simulink model "model"  (R2017a)
settings: Solver=ode45  StartTime=0.0  StopTime=2  RelTol=1e-3  EnableMultiTasking=on
undefined symbols (not defined in the file or in its folder): current_ctrl, motor, vest
libraries: simulink x1
settings Model: Creator=rodrigo  LastModifiedBy=rodrigo
settings DataIOCC: LimitDataPoints=on  SaveFormat=Array
settings OptimizationCC: LifeSpan=inf
settings DebuggingCC: UnderspecifiedInitializationDetection=Classic  MergeDetectMultiDrivingBlocksExec=none  StateNameClashWarn=warning  SFUnexpectedBacktrackingDiag=warning  SFNoUnconditionalDefaultTransitionDiag=warning  SFExecutionAtInitializationDiag=none
settings HardwareCC: ProdBitPerPointer=32  ProdBitPerSizeT=32  ProdBitPerPtrDiffT=32  ProdLargestAtomicFloat=None  ProdIntDivRoundTo=Undefined  ProdEndianess=Unspecified  ProdWordSize=32  ProdHWDeviceType=32-bit Generic
settings ModelReferenceCC: PropagateSignalLabelsOutOfModel=off
settings GRTTargetCC: TargetLangStandard=C89/C90 (ANSI)  GeneratePreprocessorConditionals=Disable all
settings ConfigComp: CovMetricSettings=dw  CovHtmlReporting=on  CovSaveCumulativeToWorkspaceVar=on  CovSaveSingleToWorkspaceVar=on  CovExternalEMLEnable=off

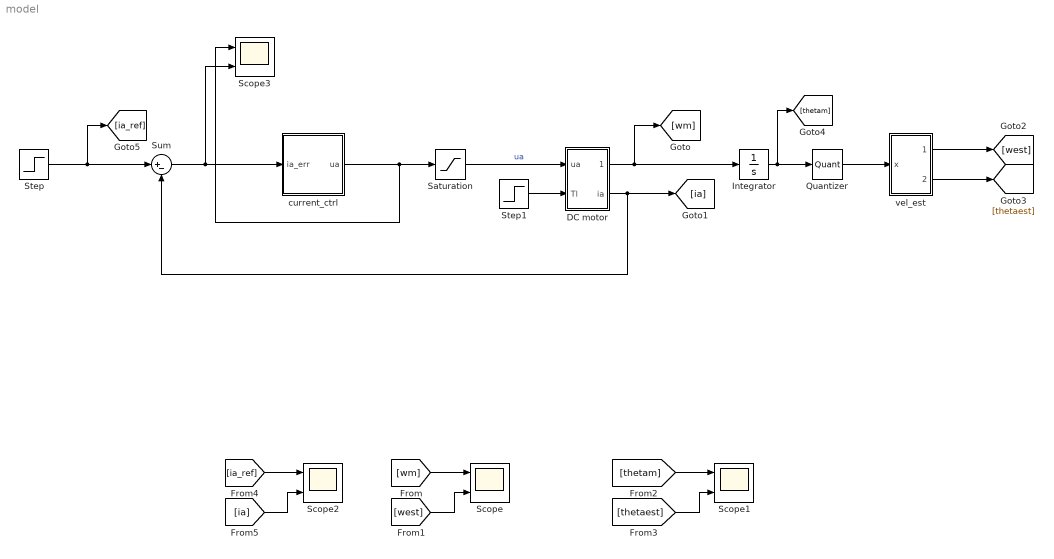
== system model ==
  DC motor : Subsystem
  Integrator : Integrator
  Quantizer : Quantizer  QuantizationInterval=encoder
  Saturation : Saturate  UpperLimit=12  LowerLimit=-12
  Scope{,1..3} (4 alike) : Scope  NumInputPorts=2
  Step : Step  Time=0.1  After=0.5  SampleTime=0
  Step1 : Step  Time=0.6  After=0.05  SampleTime=0  ZeroCross=off
  Sum : Sum  Inputs=|+-
  current_ctrl : Subsystem
  vel_est : Subsystem
  wires:
  Step/1 -> [ia_ref], Sum/1
  [wm] -> Scope/1
  [west] -> Scope/2
  DC motor/2(ia) -> [ia], Sum/2
  Step1/1 -> DC motor/2(Tl)
  Saturation/1 -> DC motor/1(ua)  "ua"
  DC motor/1(wm) -> Integrator/1, [wm]
  Integrator/1 -> [thetam], Quantizer/1
  Quantizer/1 -> vel_est/1(x)
  vel_est/1(vest) -> [west]
  [thetam] -> Scope1/1
  [thetaest] -> Scope1/2
  vel_est/2(xest) -> [thetaest]
  [ia_ref] -> Scope2/1
  [ia] -> Scope2/2
  Sum/1 -> Scope3/2, current_ctrl/1(ia_err)
  current_ctrl/1(ua) -> Scope3/1, Saturation/1

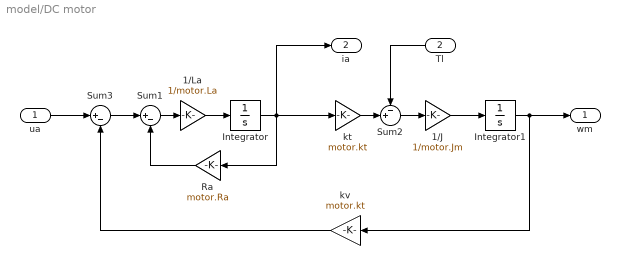
== system model/DC motor ==
  ua : Inport
  Tl : Inport  Port=2
  1/J : Gain  Gain=1/motor.Jm
  1/La : Gain  Gain=1/motor.La
  Integrator : Integrator  ZeroCross=off
  Integrator1 : Integrator
  Ra : Gain  Gain=motor.Ra
  Sum1 : Sum  Inputs=|+-
  Sum2 : Sum  Inputs=-+|
  Sum3 : Sum  Inputs=|+-
  kt : Gain  Gain=motor.kt
  kv : Gain  Gain=motor.kt
  wm : Outport
  ia : Outport  Port=2
  wires:
  1/J/1 -> Integrator1/1
  Sum2/1 -> 1/J/1
  Integrator1/1 -> wm/1, kv/1
  ua/1 -> Sum3/1
  Integrator/1 -> kt/1, Ra/1, ia/1
  Ra/1 -> Sum1/2
  1/La/1 -> Integrator/1
  Tl/1 -> Sum2/1
  kv/1 -> Sum3/2
  Sum3/1 -> Sum1/1
  kt/1 -> Sum2/2
  Sum1/1 -> 1/La/1

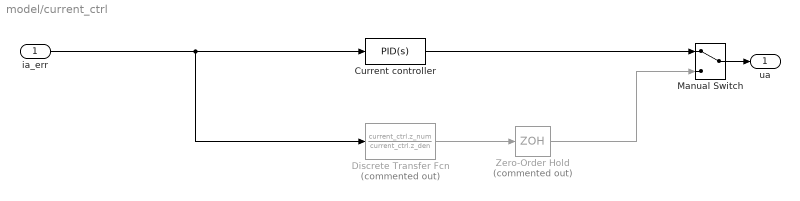
== system model/current_ctrl ==
  ia_err : Inport
  Current controller : simulink/Continuous/PID Controller  Controller=PID  TimeDomain=Continuous-time  SampleTime=-1  IntegratorMethod=Forward Euler  FilterMethod=Forward Euler  Form=Parallel  UseFilter=off  ControllerParametersSource=internal  P=current_ctrl.kp  I=current_ctrl.ki  D=0  N=100  InitialConditionSource=internal  InitialConditionForIntegrator=0  InitialConditionForFilter=0  ExternalReset=none  ZeroCross=off  LimitOutput=on  UpperSaturationLimit=12  LowerSaturationLimit=-12  LinearizeAsGain=off  AntiWindupMode=back-calculation  Kb=1  TrackingMode=off  Kt=1  PParamMin=[]  PParamMax=[]  IParamMin=[]  IParamMax=[]  DParamMin=[]  DParamMax=[]  NParamMin=[]  NParamMax=[]  KbParamMin=[]  KbParamMax=[]  KtParamMin=[]  KtParamMax=[]  POutMin=[]  POutMax=[]  IOutMin=[]  IOutMax=[]  DOutMin=[]  DOutMax=[]  NOutMin=[]  NOutMax=[]  KbOutMin=[]  KbOutMax=[]  KtOutMin=[]  KtOutMax=[]  IntegratorOutMin=[]  IntegratorOutMax=[]  FilterOutMin=[]  FilterOutMax=[]  SumOutMin=[]  SumOutMax=[]  SumI1OutMin=[]  SumI1OutMax=[]  SumI2OutMin=[]  SumI2OutMax=[]  SumI3OutMin=[]  SumI3OutMax=[]  SumDOutMin=[]  SumDOutMax=[]  SaturationOutMin=[]  SaturationOutMax=[]  IntegratorContinuousStateAttributes=''  IntegratorStateMustResolveToSignalObject=off  IntegratorRTWStateStorageClass=Auto  FilterContinuousStateAttributes=''  FilterStateMustResolveToSignalObject=off  FilterRTWStateStorageClass=Auto  DifferentiatorICPrevScaledInput=0  DifferentiatorOutMin=[]  DifferentiatorOutMax=[]  InitialConditionSetting=State (most efficient)
  Discrete Transfer Fcn : DiscreteTransferFcn  Commented=on  Numerator=current_ctrl.z_num  Denominator=current_ctrl.z_den  SampleTime=current_ctrl.Ts
  Manual Switch : ManualSwitch
  Zero-Order Hold : ZeroOrderHold  Commented=on  SampleTime=-1
  ua : Outport
  wires:
  ia_err/1 -> Discrete Transfer Fcn/1, Current controller/1
  Current controller/1 -> Manual Switch/1
  Discrete Transfer Fcn/1 -> Zero-Order Hold/1
  Zero-Order Hold/1 -> Manual Switch/2
  Manual Switch/1 -> ua/1

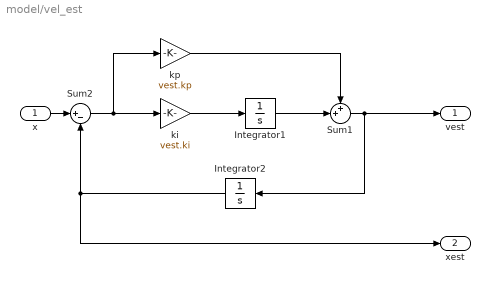
== system model/vel_est ==
  x : Inport
  Integrator1 : Integrator
  Integrator2 : Integrator
  Sum1 : Sum  Inputs=++|
  Sum2 : Sum  Inputs=|+-
  ki : Gain  Gain=vest.ki
  kp : Gain  Gain=vest.kp
  vest : Outport
  xest : Outport  Port=2
  wires:
  ki/1 -> Integrator1/1
  Sum2/1 -> kp/1, ki/1
  Integrator2/1 -> xest/1, Sum2/2
  kp/1 -> Sum1/1
  Integrator1/1 -> Sum1/2
  x/1 -> Sum2/1
  Sum1/1 -> vest/1, Integrator2/1
